simulink subsystem "foc_sensorless_algorithm"  (R2021b)
settings: Solver=VariableStepAuto  StartTime=0.0  StopTime=10.0  RelTol=1e-3
values from neighbouring files (symbols this model uses):
  PI_params = mcb.internal.SetControllerParameters(pmsm,inverter,PU_System,T_pwm,2*Ts,Ts_speed)    [mcb_pmsm_foc_dual_f28379d_data.m]    (also in mcb_pmsm_foc_dual_f28379d_datascript.m; mcb_pmsm_foc_f280049C_data.m = mcb.internal.SetControllerParameters(pmsm,inverter,PU_System; mcb_pmsm_foc_f28335_data.m = mcb.internal.SetControllerParameters(pmsm,inverter,PU_System; mcb_pmsm_foc_hall_f28035_data.m = mcb.internal.SetControllerParameters(pmsm,inverter,PU_System)
  pmsm = struct    [c28335_pmsmfoc_data.m]    (also in mcb_pmsm_foc_dual_f28379d_data.m = mcb_SetPMSMMotorParameters('Teknic2310P'); mcb_pmsm_foc_dual_f28379d_datascript.m = mcb_SetPMSMMotorParameters('Teknic2310P'); mcb_pmsm_foc_f280049C_data.m = mcb_SetPMSMMotorParameters('BLY171D'); mcb_pmsm_foc_f28335_data.m = mcb_SetPMSMMotorParameters('BLY171D'))
  PU_System = mcb_SetPUSystem(pmsm,inverter)    [mcb_pmsm_foc_dual_f28379d_data.m]    (also in mcb_pmsm_foc_dual_f28379d_datascript.m; mcb_pmsm_foc_f280049C_data.m; mcb_pmsm_foc_f28335_data.m; mcb_pmsm_foc_hall_f28035_data.m)
  Speed_openLoop_PU = 0.1    [mcb_pmsm_foc_dual_f28379d_data.m]    (also in mcb_pmsm_foc_dual_f28379d_datascript.m; mcb_pmsm_foc_sensorless_dyno_f28379d_data.m; mcb_pmsm_foc_sensorless_dyno_f28379d_datascript.m; mcb_pmsm_foc_sensorless_f280049C_data.m)
  Ts = 5e-8    (= 5e-08)    [DCDC_Buck_Param.m]    (also in mcb_c2000_open_loop_control_data.m = T_pwm; mcb_c2000_pmsm_offset_data.m = T_pwm; mcb_pmsm_foc_dual_f28379d_data.m = 5e-05; mcb_pmsm_foc_dual_f28379d_datascript.m = 5e-05)
  Ts_speed = 20*Ts    (= 0.001)    [mcb_pmsm_foc_dual_f28379d_data.m]    (also in mcb_pmsm_foc_dual_f28379d_datascript.m; mcb_pmsm_foc_f280049C_data.m = 0.0005; mcb_pmsm_foc_f28335_data.m = 0.0005; mcb_pmsm_foc_hall_f28035_data.m = 0.0005)
libraries: mcbcontrolslib x11
settings Model: Creator=The MathWorks, Inc.  LastModifiedBy=The MathWorks, Inc.
settings SolverCC: AlgebraicLoopSolver=TrustRegion
settings DebuggingCC: SFMachineParentedDataDiag=warning

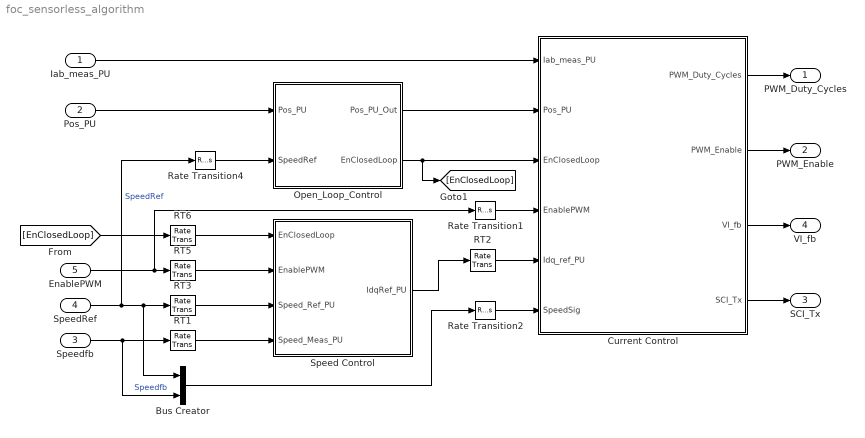
== system foc_sensorless_algorithm ==
  Iab_meas_PU : Inport
  Pos_PU : Inport  Port=2
  Speedfb : Inport  Port=3
  SpeedRef : Inport  Port=4
  EnablePWM : Inport  Port=5
  Bus Creator : BusCreator  Inputs=2
  Current Control : Subsystem  TreatAsAtomicUnit=on
      settings: RTWSystemCode=Nonreusable function
  Open_Loop_Control : Subsystem  TreatAsAtomicUnit=on
      settings: RTWSystemCode=Nonreusable function
  RT{1,3,5..6} (4 alike) : RateTransition  Deterministic=off  OutPortSampleTime=Ts_speed
  RT2 : RateTransition  Deterministic=off
  Rate Transition1 : RateTransition  Deterministic=off
  Rate Transition2 : RateTransition  Deterministic=off
  Rate Transition4 : RateTransition  Deterministic=off
  Speed Control : Subsystem  TreatAsAtomicUnit=on  SystemSampleTime=Ts_speed
  PWM_Duty_Cycles : Outport
  PWM_Enable : Outport  Port=2
  SCI_Tx : Outport  Port=3
  VI_fb : Outport  Port=4
  wires:
  RT1/1 -> Speed Control/4(Speed_Meas_PU)
  Current Control/1(PWM_Duty_Cycles) -> PWM_Duty_Cycles/1
  Open_Loop_Control/2(EnClosedLoop) -> [EnClosedLoop], Current Control/3(EnClosedLoop)
  Open_Loop_Control/1(Pos_PU_Out) -> Current Control/2(Pos_PU)
  Speed Control/1(IdqRef_PU) -> RT2/1
  RT2/1 -> Current Control/5(Idq_ref_PU)
  RT3/1 -> Speed Control/3(Speed_Ref_PU)
  RT5/1 -> Speed Control/2(EnablePWM)
  RT6/1 -> Speed Control/1(EnClosedLoop)
  SpeedRef/1 -> RT3/1, Bus Creator/1, Rate Transition4/1  "SpeedRef"
  Speedfb/1 -> RT1/1, Bus Creator/2  "Speedfb"
  Current Control/2(PWM_Enable) -> PWM_Enable/1
  Pos_PU/1 -> Open_Loop_Control/1(Pos_PU)
  [EnClosedLoop] -> RT6/1
  Iab_meas_PU/1 -> Current Control/1(Iab_meas_PU)
  Current Control/3(VI_fb) -> VI_fb/1
  Current Control/4(SCI_Tx) -> SCI_Tx/1
  EnablePWM/1 -> RT5/1, Rate Transition1/1
  Bus Creator/1 -> Rate Transition2/1
  Rate Transition4/1 -> Open_Loop_Control/2(SpeedRef)
  Rate Transition1/1 -> Current Control/4(EnablePWM)
  Rate Transition2/1 -> Current Control/6(SpeedSig)

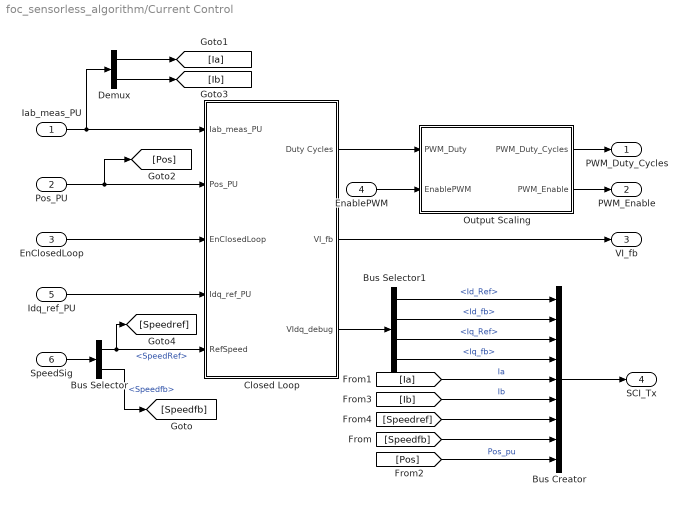
== system foc_sensorless_algorithm/Current Control ==
  Iab_meas_PU : Inport
  Pos_PU : Inport  Port=2
  EnClosedLoop : Inport  Port=3
  EnablePWM : Inport  Port=4
  Idq_ref_PU : Inport  Port=5
  SpeedSig : Inport  Port=6
  Bus Creator : BusCreator  Inputs=9
  Bus Selector : BusSelector  OutputSignals=SpeedRef,Speedfb
  Bus Selector1 : BusSelector  OutputSignals=Id_Ref,Id_fb,Iq_Ref,Iq_fb
  Closed Loop : Subsystem
  Demux : Demux  Outputs=2
  Output Scaling : Subsystem
  PWM_Duty_Cycles : Outport
  PWM_Enable : Outport  Port=2
  VI_fb : Outport  Port=3
  SCI_Tx : Outport  Port=4
  wires:
  Bus Selector/1 -> [Speedref], Closed Loop/5(RefSpeed)  "<SpeedRef>"
  SpeedSig/1 -> Bus Selector/1
  EnClosedLoop/1 -> Closed Loop/3(EnClosedLoop)
  EnablePWM/1 -> Output Scaling/2(EnablePWM)
  Closed Loop/3(VIdq_debug) -> Bus Selector1/1
  Output Scaling/1(PWM_Duty_Cycles) -> PWM_Duty_Cycles/1
  Closed Loop/2(VI_fb) -> VI_fb/1
  Closed Loop/1(Duty Cycles) -> Output Scaling/1(PWM_Duty)
  Idq_ref_PU/1 -> Closed Loop/4(Idq_ref_PU)
  Pos_PU/1 -> [Pos], Closed Loop/2(Pos_PU)
  Output Scaling/2(PWM_Enable) -> PWM_Enable/1
  Iab_meas_PU/1 -> Demux/1, Closed Loop/1(Iab_meas_PU)
  Bus Creator/1 -> SCI_Tx/1
  Bus Selector/2 -> [Speedfb]  "<Speedfb>"
  Demux/1 -> [Ia]
  Demux/2 -> [Ib]
  Bus Selector1/2 -> Bus Creator/2  "<Id_fb>"
  Bus Selector1/4 -> Bus Creator/4  "<Iq_fb>"
  [Speedfb] -> Bus Creator/8
  [Ia] -> Bus Creator/5  "Ia"
  [Pos] -> Bus Creator/9  "Pos_pu"
  Bus Selector1/1 -> Bus Creator/1  "<Id_Ref>"
  Bus Selector1/3 -> Bus Creator/3  "<Iq_Ref>"
  [Ib] -> Bus Creator/6  "Ib"
  [Speedref] -> Bus Creator/7

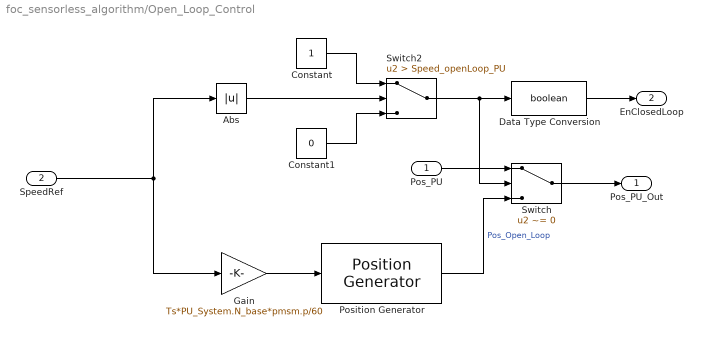
== system foc_sensorless_algorithm/Open_Loop_Control ==
  Pos_PU : Inport
  SpeedRef : Inport  Port=2
  Abs : Abs
  Constant : Constant  OutDataTypeStr=uint16
  Constant1 : Constant  Value=0  OutDataTypeStr=uint16
  Data Type Conversion : DataTypeConversion  OutDataTypeStr=boolean  RndMeth=Simplest
  Gain : Gain  Gain=Ts*PU_System.N_base*pmsm.p/60  OutDataTypeStr=Inherit: Same as input  ParamDataTypeStr=Inherit: Same as input
  Position Generator : mcbcontrolslib/Position Generator  AngleOutput=Per-unit  ThetaSource=External  ThetaInput=5e-4  DataType=double  ExternalReset=none  Offset=0
      settings: SourceProductBaseCode=MT
  Switch : Switch  Criteria=u2 ~= 0  Threshold=0.1
  Switch2 : Switch  Criteria=u2 > Threshold  Threshold=Speed_openLoop_PU
  Pos_PU_Out : Outport
  EnClosedLoop : Outport  Port=2
  wires:
  Position Generator/1 -> Switch/3  "Pos_Open_Loop"
  Data Type Conversion/1 -> EnClosedLoop/1
  SpeedRef/1 -> Gain/1, Abs/1
  Switch2/1 -> Data Type Conversion/1, Switch/2
  Gain/1 -> Position Generator/1
  Switch/1 -> Pos_PU_Out/1
  Pos_PU/1 -> Switch/1
  Abs/1 -> Switch2/2
  Constant/1 -> Switch2/1
  Constant1/1 -> Switch2/3

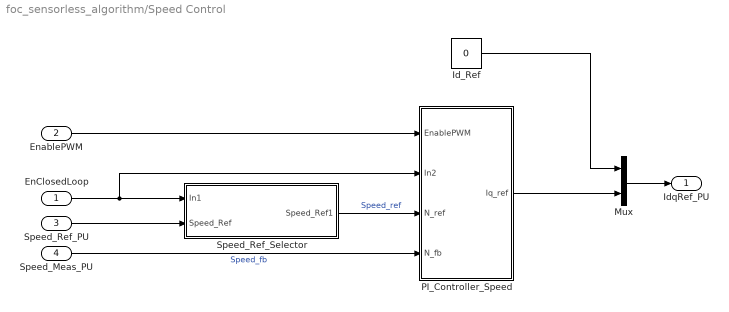
== system foc_sensorless_algorithm/Speed Control ==
  EnClosedLoop : Inport
  EnablePWM : Inport  Port=2
  Speed_Ref_PU : Inport  Port=3
  Speed_Meas_PU : Inport  Port=4
  Id_Ref : Constant  Value=0  OutDataTypeStr=dataType
  Mux : Mux  Inputs=2
  PI_Controller_Speed : Subsystem
  Speed_Ref_Selector : Subsystem
  IdqRef_PU : Outport  VectorParamsAs1DForOutWhenUnconnected=off
  wires:
  EnablePWM/1 -> PI_Controller_Speed/1(EnablePWM)
  EnClosedLoop/1 -> Speed_Ref_Selector/1(In1), PI_Controller_Speed/2(In2)
  Speed_Ref_Selector/1(Speed_Ref1) -> PI_Controller_Speed/3(N_ref)  "Speed_ref"
  Speed_Ref_PU/1 -> Speed_Ref_Selector/2(Speed_Ref)
  Mux/1 -> IdqRef_PU/1
  Id_Ref/1 -> Mux/1
  Speed_Meas_PU/1 -> PI_Controller_Speed/4(N_fb)  "Speed_fb"
  PI_Controller_Speed/1(Iq_ref) -> Mux/2

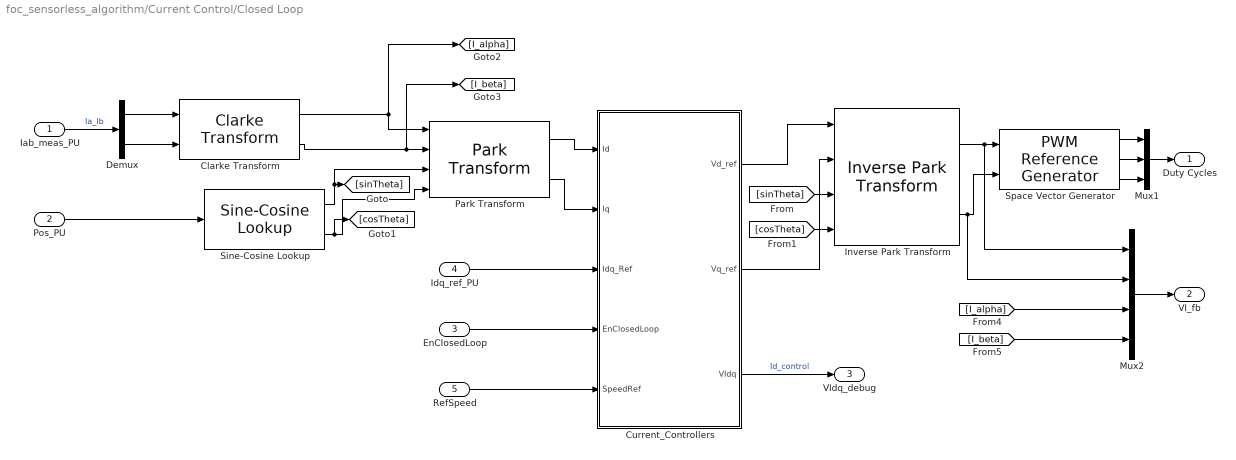
== system foc_sensorless_algorithm/Current Control/Closed Loop ==
  Iab_meas_PU : Inport
  Pos_PU : Inport  Port=2
  EnClosedLoop : Inport  Port=3
  Idq_ref_PU : Inport  Port=4
  RefSpeed : Inport  Port=5
  Clarke Transform : mcbcontrolslib/Clarke Transform  VariantControl=Variant2
  Current_Controllers : Subsystem
  Demux : Demux  Outputs=2
  Inverse Park Transform : mcbcontrolslib/Inverse Park Transform  AxisAlignment=D-axis
  Mux1 : Mux  Inputs=3
  Mux2 : Mux
  Park Transform : mcbcontrolslib/Park Transform  AxisAlignment=D-axis
      settings: SourceProductBaseCode=MT
  Sine-Cosine Lookup : mcbcontrolslib/Sine-Cosine Lookup  AngleInput=Per-unit  N_points=1024
      settings: SourceProductBaseCode=MT
  Space Vector Generator : mcbcontrolslib/PWM Reference Generator  inSignal=Valphabeta  modType=SVM: space vector modulation
      settings: SourceProductBaseCode=MT
  Duty Cycles : Outport  VectorParamsAs1DForOutWhenUnconnected=off
  VI_fb : Outport  Port=2  VectorParamsAs1DForOutWhenUnconnected=off
  VIdq_debug : Outport  Port=3  VectorParamsAs1DForOutWhenUnconnected=off
  wires:
  RefSpeed/1 -> Current_Controllers/5(SpeedRef)
  EnClosedLoop/1 -> Current_Controllers/4(EnClosedLoop)
  Pos_PU/1 -> Sine-Cosine Lookup/1
  Current_Controllers/3(VIdq) -> VIdq_debug/1  "Id_control"
  Idq_ref_PU/1 -> Current_Controllers/3(Idq_Ref)
  Iab_meas_PU/1 -> Demux/1  "Ia_Ib"
  Demux/2 -> Clarke Transform/2
  Demux/1 -> Clarke Transform/1
  Park Transform/2 -> Current_Controllers/2(Iq)
  Park Transform/1 -> Current_Controllers/1(Id)
  Space Vector Generator/2 -> Mux1/2
  Sine-Cosine Lookup/2 -> [cosTheta], Park Transform/4
  Mux1/1 -> Duty Cycles/1
  Space Vector Generator/3 -> Mux1/3
  Space Vector Generator/1 -> Mux1/1
  [I_alpha] -> Mux2/3
  Sine-Cosine Lookup/1 -> Park Transform/3, [sinTheta]
  Clarke Transform/2 -> Park Transform/2, [I_beta]
  Current_Controllers/2(Vq_ref) -> Inverse Park Transform/2
  Clarke Transform/1 -> [I_alpha], Park Transform/1
  Mux2/1 -> VI_fb/1
  [sinTheta] -> Inverse Park Transform/3
  Inverse Park Transform/1 -> Space Vector Generator/1, Mux2/1
  Inverse Park Transform/2 -> Mux2/2, Space Vector Generator/2
  [I_beta] -> Mux2/4
  [cosTheta] -> Inverse Park Transform/4
  Current_Controllers/1(Vd_ref) -> Inverse Park Transform/1

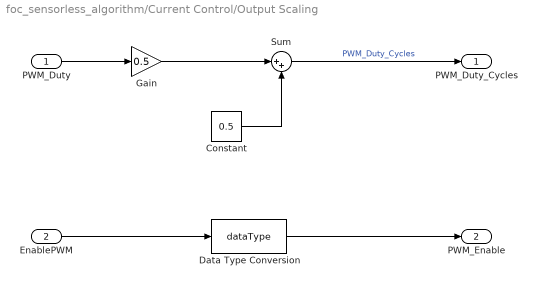
== system foc_sensorless_algorithm/Current Control/Output Scaling ==
  PWM_Duty : Inport
  EnablePWM : Inport  Port=2
  Constant : Constant  Value=0.5  OutDataTypeStr=dataType
  Data Type Conversion : DataTypeConversion  OutDataTypeStr=dataType
  Gain : Gain  Gain=0.5  OutDataTypeStr=Inherit: Same as input
  Sum : Sum  Inputs=|++
  PWM_Duty_Cycles : Outport
  PWM_Enable : Outport  Port=2
  wires:
  EnablePWM/1 -> Data Type Conversion/1
  Data Type Conversion/1 -> PWM_Enable/1
  PWM_Duty/1 -> Gain/1
  Gain/1 -> Sum/1
  Constant/1 -> Sum/2
  Sum/1 -> PWM_Duty_Cycles/1  "PWM_Duty_Cycles"

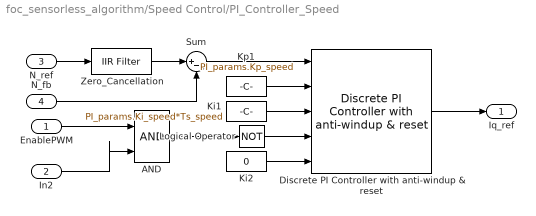
== system foc_sensorless_algorithm/Speed Control/PI_Controller_Speed ==
  EnablePWM : Inport
  In2 : Inport  Port=2
  N_ref : Inport  Port=3
  N_fb : Inport  Port=4
  AND : Logic  IconShape=distinctive  AllPortsSameDT=off  OutDataTypeStr=boolean
  Discrete PI Controller with anti-windup & reset : mcbcontrolslib/Discrete PI Controller  with anti-windup & reset  UpperSaturationLimit=1  LowerSaturationLimit=-1
      settings: SourceProductBaseCode=MT
  Ki1 : Constant  Value=PI_params.Ki_speed*Ts_speed  OutDataTypeStr=dataType  SampleTime=-1
  Ki2 : Constant  Value=0  OutDataTypeStr=dataType  SampleTime=-1
  Kp1 : Constant  Value=PI_params.Kp_speed  OutDataTypeStr=dataType  SampleTime=-1
  Logical Operator : Logic  Operator=NOT  IconShape=distinctive  AllPortsSameDT=off  OutDataTypeStr=boolean
  Sum : Sum  Inputs=|+-  OutDataTypeStr=Inherit: Same as first input
  Zero_Cancellation : mcbcontrolslib/IIR Filter  VariantControl=Low Pass Filter  VariantSelect=Low-pass  Filter_constant=0.01*(Ts_speed/Ts)  advancedSettings=off  Ts=50e-6  cutOff_freq=1
      settings: SourceProductBaseCode=MT
  Iq_ref : Outport  VectorParamsAs1DForOutWhenUnconnected=off
  wires:
  Zero_Cancellation/1 -> Sum/1
  AND/1 -> Logical Operator/1
  In2/1 -> AND/2
  EnablePWM/1 -> AND/1
  Ki2/1 -> Discrete PI Controller with anti-windup & reset/5
  Logical Operator/1 -> Discrete PI Controller with anti-windup & reset/4
  Sum/1 -> Discrete PI Controller with anti-windup & reset/1
  N_ref/1 -> Zero_Cancellation/1
  N_fb/1 -> Sum/2
  Kp1/1 -> Discrete PI Controller with anti-windup & reset/2
  Ki1/1 -> Discrete PI Controller with anti-windup & reset/3
  Discrete PI Controller with anti-windup & reset/1 -> Iq_ref/1

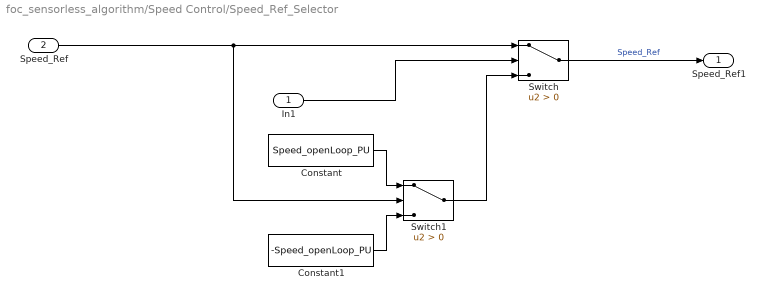
== system foc_sensorless_algorithm/Speed Control/Speed_Ref_Selector ==
  In1 : Inport
  Speed_Ref : Inport  Port=2
  Constant : Constant  Value=Speed_openLoop_PU  OutDataTypeStr=dataType
  Constant1 : Constant  Value=-Speed_openLoop_PU  OutDataTypeStr=dataType
  Switch : Switch  Criteria=u2 > Threshold
  Switch1 : Switch  Criteria=u2 > Threshold
  Speed_Ref1 : Outport
  wires:
  Constant1/1 -> Switch1/3
  Switch1/1 -> Switch/3
  Constant/1 -> Switch1/1
  Switch/1 -> Speed_Ref1/1  "Speed_Ref"
  In1/1 -> Switch/2
  Speed_Ref/1 -> Switch/1, Switch1/2

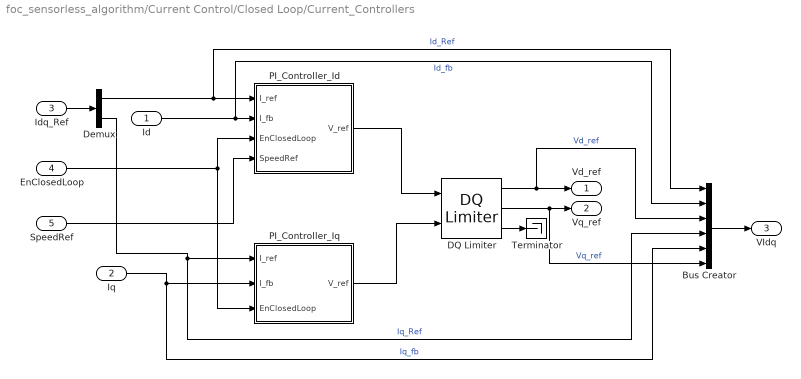
== system foc_sensorless_algorithm/Current Control/Closed Loop/Current_Controllers ==
  Id : Inport
  Iq : Inport  Port=2
  Idq_Ref : Inport  Port=3
  EnClosedLoop : Inport  Port=4
  SpeedRef : Inport  Port=5
  Bus Creator : BusCreator  Inputs=6
  DQ Limiter : mcbcontrolslib/DQ Limiter  Vmax=0.95
      settings: SourceProductBaseCode=MT
  Demux : Demux  Outputs=2
  PI_Controller_Id : Subsystem
  PI_Controller_Iq : Subsystem
  Terminator : Terminator
  Vd_ref : Outport  VectorParamsAs1DForOutWhenUnconnected=off
  Vq_ref : Outport  Port=2  VectorParamsAs1DForOutWhenUnconnected=off
  VIdq : Outport  Port=3  VectorParamsAs1DForOutWhenUnconnected=off
  wires:
  DQ Limiter/1 -> Vd_ref/1, Bus Creator/3  "Vd_ref"
  Demux/1 -> PI_Controller_Id/1(I_ref), Bus Creator/1  "Id_Ref"
  Iq/1 -> Bus Creator/5, PI_Controller_Iq/2(I_fb)  "Iq_fb"
  DQ Limiter/2 -> Bus Creator/6, Vq_ref/1  "Vq_ref"
  Demux/2 -> Bus Creator/4, PI_Controller_Iq/1(I_ref)  "Iq_Ref"
  Bus Creator/1 -> VIdq/1
  SpeedRef/1 -> PI_Controller_Id/4(SpeedRef)
  EnClosedLoop/1 -> PI_Controller_Iq/3(EnClosedLoop), PI_Controller_Id/3(EnClosedLoop)
  Idq_Ref/1 -> Demux/1
  DQ Limiter/3 -> Terminator/1
  PI_Controller_Iq/1(V_ref) -> DQ Limiter/2
  Id/1 -> PI_Controller_Id/2(I_fb), Bus Creator/2  "Id_fb"
  PI_Controller_Id/1(V_ref) -> DQ Limiter/1

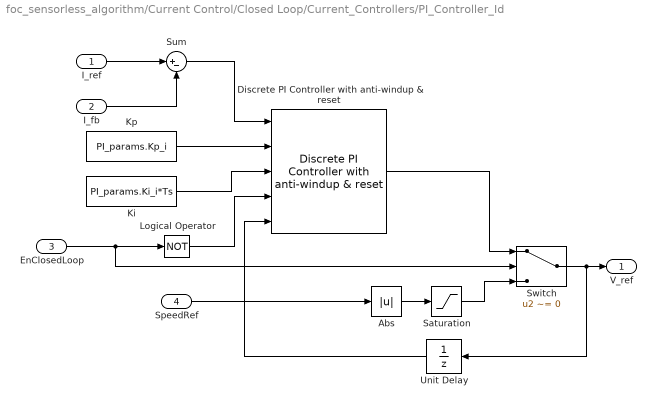
== system foc_sensorless_algorithm/Current Control/Closed Loop/Current_Controllers/PI_Controller_Id ==
  I_ref : Inport
  I_fb : Inport  Port=2
  EnClosedLoop : Inport  Port=3
  SpeedRef : Inport  Port=4
  Abs : Abs  RndMeth=Simplest
  Discrete PI Controller with anti-windup & reset : mcbcontrolslib/Discrete PI Controller  with anti-windup & reset  UpperSaturationLimit=1  LowerSaturationLimit=-1
      settings: SourceProductBaseCode=MT
  Ki : Constant  Value=PI_params.Ki_i*Ts  OutDataTypeStr=dataType  SampleTime=-1
  Kp : Constant  Value=PI_params.Kp_i  OutDataTypeStr=dataType  SampleTime=-1
  Logical Operator : Logic  Operator=NOT  IconShape=distinctive  AllPortsSameDT=off  OutDataTypeStr=boolean
  Saturation : Saturate  LowerLimit=0.15  RndMeth=Simplest
  Sum : Sum  Inputs=|+-  OutDataTypeStr=Inherit: Same as first input
  Switch : Switch  Criteria=u2 ~= 0  RndMeth=Simplest
  Unit Delay : UnitDelay  SampleTime=-1  HasFrameUpgradeWarning=on
  V_ref : Outport  VectorParamsAs1DForOutWhenUnconnected=off
  wires:
  Saturation/1 -> Switch/3
  SpeedRef/1 -> Abs/1
  Abs/1 -> Saturation/1
  EnClosedLoop/1 -> Switch/2, Logical Operator/1
  Discrete PI Controller with anti-windup & reset/1 -> Switch/1
  Unit Delay/1 -> Discrete PI Controller with anti-windup & reset/5
  Logical Operator/1 -> Discrete PI Controller with anti-windup & reset/4
  Ki/1 -> Discrete PI Controller with anti-windup & reset/3
  I_ref/1 -> Sum/1
  Kp/1 -> Discrete PI Controller with anti-windup & reset/2
  Sum/1 -> Discrete PI Controller with anti-windup & reset/1
  I_fb/1 -> Sum/2
  Switch/1 -> Unit Delay/1, V_ref/1

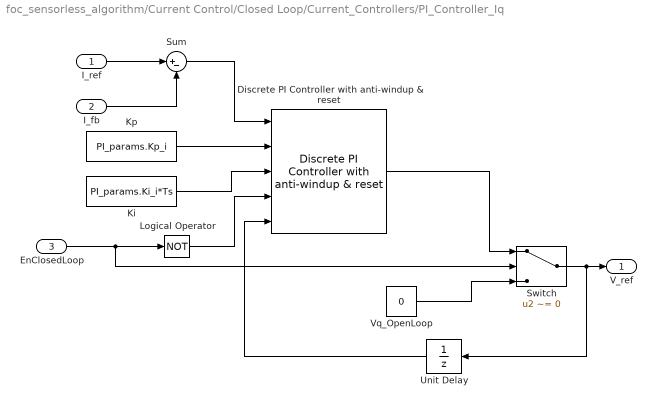
== system foc_sensorless_algorithm/Current Control/Closed Loop/Current_Controllers/PI_Controller_Iq ==
  I_ref : Inport
  I_fb : Inport  Port=2
  EnClosedLoop : Inport  Port=3
  Discrete PI Controller with anti-windup & reset : mcbcontrolslib/Discrete PI Controller  with anti-windup & reset  UpperSaturationLimit=1  LowerSaturationLimit=-1
      settings: SourceProductBaseCode=MT
  Ki : Constant  Value=PI_params.Ki_i*Ts  OutDataTypeStr=dataType  SampleTime=-1
  Kp : Constant  Value=PI_params.Kp_i  OutDataTypeStr=dataType  SampleTime=-1
  Logical Operator : Logic  Operator=NOT  IconShape=distinctive  AllPortsSameDT=off  OutDataTypeStr=boolean
  Sum : Sum  Inputs=|+-  OutDataTypeStr=Inherit: Same as first input
  Switch : Switch  Criteria=u2 ~= 0  RndMeth=Simplest
  Unit Delay : UnitDelay  SampleTime=-1  HasFrameUpgradeWarning=on
  Vq_OpenLoop : Constant  Value=0  OutDataTypeStr=dataType  SampleTime=-1
  V_ref : Outport  VectorParamsAs1DForOutWhenUnconnected=off
  wires:
  EnClosedLoop/1 -> Switch/2, Logical Operator/1
  Vq_OpenLoop/1 -> Switch/3
  Discrete PI Controller with anti-windup & reset/1 -> Switch/1
  Unit Delay/1 -> Discrete PI Controller with anti-windup & reset/5
  Logical Operator/1 -> Discrete PI Controller with anti-windup & reset/4
  Ki/1 -> Discrete PI Controller with anti-windup & reset/3
  I_ref/1 -> Sum/1
  Kp/1 -> Discrete PI Controller with anti-windup & reset/2
  Sum/1 -> Discrete PI Controller with anti-windup & reset/1
  I_fb/1 -> Sum/2
  Switch/1 -> Unit Delay/1, V_ref/1
